simulink model "parte3_eje6_avr_stb4"  (R2017b)
settings: Solver=VariableStepAuto  StartTime=0.0  StopTime=200  RelTol=1e-3
values from neighbouring files (symbols this model uses):
  aKp = 6.73    [parte3_eje5_ESSTB.m]
  IFDfin = 1000    [parte3_eje3_EXAC1.m]    (also in parte3_eje3_EXAC2.m = 0; parte3_eje5_ESSTB.m = 1)
  KC = 0.2    [parte3_eje3_EXAC1.m]    (also in parte3_eje3_EXAC2.m; parte3_eje5_ESSTB.m = 0.1; parte3_eje6_ESST1A.m = 0.01)
  KG = 0.1    [parte3_eje5_ESSTB.m]
  KI = 0.1    [parte3_eje5_ESSTB.m]
  KIM = 0.2    [parte3_eje5_ESSTB.m]
  KIR = 2.97    [parte3_eje5_ESSTB.m]
  KPM = 1    [parte3_eje5_ESSTB.m]
  KPR = 2.97    [parte3_eje5_ESSTB.m]
  Ta = 0.02    [parte3_eje3_EXAC1.m]    (also in parte3_eje3_EXAC2.m; parte3_eje5_ESSTB.m = 0.01)
  VMMAX = 1    [parte3_eje5_ESSTB.m]
  VMMIN = -0.87    [parte3_eje5_ESSTB.m]
  Vrefin = 1    [parte3_eje3_EXAC1.m]    (also in parte3_eje3_EXAC2.m; parte3_eje5_ESSTB.m = 0.01)
  VRMAX = 1.7    [parte3_DC1A_data.m]    (also in parte3_eje5_ESSTB.m = 1; parte3_eje6_ESST1A.m = 3.4)
  VRMIN = -1.7    [parte3_DC1A_data.m]    (also in parte3_eje5_ESSTB.m = -0.87; parte3_eje6_ESST1A.m = -3.4)
  XL = 0    [parte3_eje5_ESSTB.m]
settings Model: Creator=cjuar  LastModifiedBy=cjuar

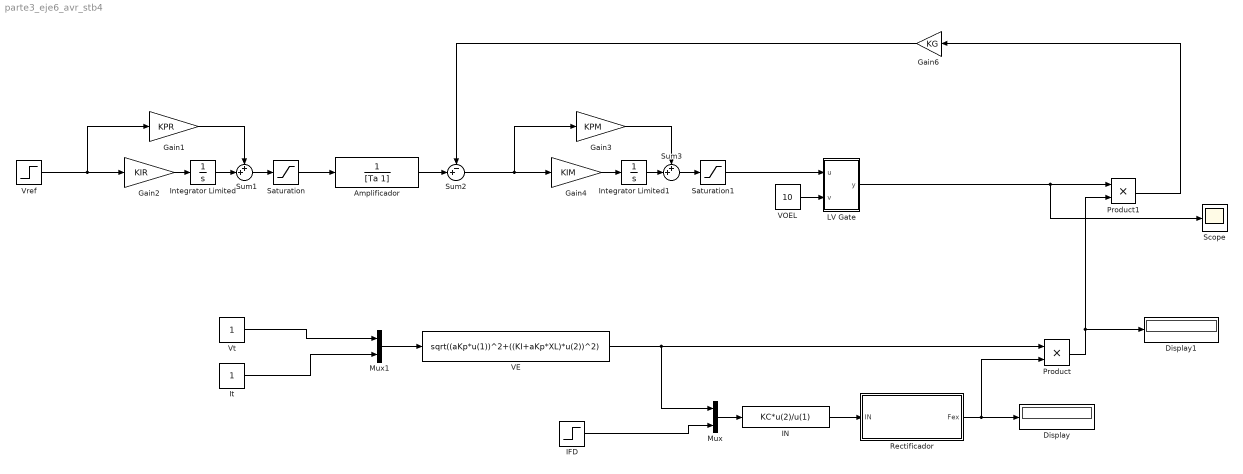
== system parte3_eje6_avr_stb4 ==
  Amplificador : TransferFcn  Denominator=[Ta 1]
  Display : Display
  Display1 : Display
  Gain1 : Gain  Gain=KPR
  Gain2 : Gain  Gain=KIR
  Gain3 : Gain  Gain=KPM
  Gain4 : Gain  Gain=KIM
  Gain6 : Gain  Gain=KG
  IFD : Step  After=IFDfin  SampleTime=0
  IN : Fcn  Expr=KC*u(2)/u(1)
  Integrator Limited : Integrator  LimitOutput=on  UpperSaturationLimit=VRMAX  LowerSaturationLimit=VRMIN
  Integrator Limited1 : Integrator  LimitOutput=on  UpperSaturationLimit=VMMAX  LowerSaturationLimit=VMMIN
  It : Constant
  LV Gate : Subsystem
  Mux : Mux  Inputs=2
  Mux1 : Mux  Inputs=2
  Product : Product
  Product1 : Product
  Rectificador : MATLAB Function  TreatAsAtomicUnit=on
  Saturation : Saturate  UpperLimit=VRMAX  LowerLimit=VRMIN
  Saturation1 : Saturate  UpperLimit=VMMAX  LowerLimit=VMMIN
  Scope : Scope
  Sum1 : Sum  Inputs=++|
  Sum2 : Sum  Inputs=-+|
  Sum3 : Sum  Inputs=++|
  VE : Fcn  Expr=sqrt((aKp*u(1))^2+((KI+aKp*XL)*u(2))^2)
  VOEL : Constant  Value=10
  Vref : Step  After=Vrefin  SampleTime=0
  Vt : Constant
  wires:
  Product/1 -> Display1/1, Product1/2
  Vref/1 -> Gain1/1, Gain2/1
  Mux/1 -> IN/1
  IN/1 -> Rectificador/1(IN)
  IFD/1 -> Mux/2
  Rectificador/1(Fex) -> Product/2, Display/1
  Amplificador/1 -> Sum2/2
  Gain6/1 -> Sum2/1
  Saturation1/1 -> LV Gate/1(u)
  VOEL/1 -> LV Gate/2(v)
  Mux1/1 -> VE/1
  Vt/1 -> Mux1/1
  It/1 -> Mux1/2
  VE/1 -> Mux/1, Product/1
  Product1/1 -> Gain6/1
  LV Gate/1(y) -> Scope/1, Product1/1
  Gain2/1 -> Integrator Limited/1
  Gain1/1 -> Sum1/1
  Integrator Limited/1 -> Sum1/2
  Sum1/1 -> Saturation/1
  Sum3/1 -> Saturation1/1
  Gain3/1 -> Sum3/1
  Integrator Limited1/1 -> Sum3/2
  Gain4/1 -> Integrator Limited1/1
  Sum2/1 -> Gain3/1, Gain4/1
  Saturation/1 -> Amplificador/1

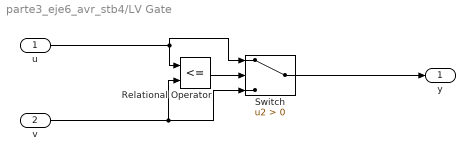
== system parte3_eje6_avr_stb4/LV Gate ==
  u : Inport
  v : Inport  Port=2
  Relational Operator : RelationalOperator  Operator=<=  OutDataTypeStr=boolean  RndMeth=Simplest
  Switch : Switch  Criteria=u2 > Threshold  InputSameDT=on
  y : Outport
  wires:
  u/1 -> Switch/1, Relational Operator/1
  Switch/1 -> y/1
  v/1 -> Switch/3, Relational Operator/2
  Relational Operator/1 -> Switch/2

== matlab function parte3_eje6_avr_stb4/Rectificador ==
  data: IN input; Fex output
function Fex = Rectificador(IN)
if IN<=0
    Fex=1;
elseif IN<=0.433
    Fex=1-0.577*IN;
elseif IN>0.433&&IN<0.75
    Fex=sqrt(0.75-IN^2);
elseif IN>=0.75&&IN<=1
    Fex=1.732*(1-IN);
else
    Fex=0;
end
